simulink model "pendule"  (R2012b)
settings: Solver=ode45  StartTime=0.0  StopTime=10  MaxStep=10  RelTol=1e-3  AbsTol=1e-3
settings Model: ExtModeTrigMode=oneshot  ExtModeArmWhenConnect=off  Creator=ArbenCela  LastModifiedBy=lalinden
settings DataIOCC: LimitDataPoints=off  SignalLoggingSaveFormat=ModelDataLogs  SaveOutput=off  SaveTime=off
settings OptimizationCC: BlockReduction=off  BooleanDataType=off  ExpressionDepthLimit=128  InitFltsAndDblsToZero=on
settings DebuggingCC: SaveWithParameterizedLinksMsg=none  SignalResolutionControl=TryResolveAllWithWarning  SolverPrmCheckMsg=none  MultiTaskDSMMsg=warning  MultiTaskCondExecSysMsg=none  FcnCallInpInsideContextMsg=UseLocalSettings  StateNameClashWarn=none  StrictBusMsg=None
settings HardwareCC: TargetUnknown=on
settings RTWCC: IncludeERTFirstTime=on
settings CodeAppCC: CustomSymbolStrType=$N$R$M_T  InternalIdentifier=Shortened
settings GRTTargetCC: TargetFcnLib=ansi_tfl_tmw.mat  CodeReplacementLibrary=None  CombineOutputUpdateFcns=off  CPPClassGenCompliant=on  GRTInterface=on

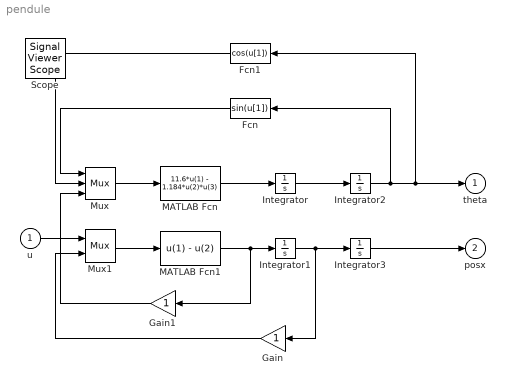
== system pendule ==
  u : Inport
  Fcn : Fcn
  Fcn1 : Fcn  Expr=cos(u[1])
  Gain : Gain  SaturateOnIntegerOverflow=on  OutDataTypeStr=Inherit: Same as input  ParamDataTypeStr=Inherit: Same as input
  Gain1 : Gain  SaturateOnIntegerOverflow=on  OutDataTypeStr=Inherit: Same as input  ParamDataTypeStr=Inherit: Same as input
  Integrator{,1..3} (4 alike) : Integrator
  MATLAB Fcn : MATLABFcn  MATLABFcn=11.6*u(1) - 1.184*u(2)*u(3)  OutputDimensions=1
  MATLAB Fcn1 : MATLABFcn  MATLABFcn=u(1) - u(2)  OutputDimensions=1
  Mux : Mux  Inputs=3
  Mux1 : Mux  Inputs=2
  theta : Outport
  posx : Outport  Port=2
  Scope : SignalViewerScope  IOType=viewer  RefreshTime=0.035000
  wires:
  u/1 -> Mux1/1
  Gain/1 -> Mux1/2
  Gain1/1 -> Mux/3
  MATLAB Fcn1/1 -> Gain1/1, Integrator1/1
  MATLAB Fcn/1 -> Integrator/1
  Mux/1 -> MATLAB Fcn/1
  Mux1/1 -> MATLAB Fcn1/1
  Fcn1/1 -> Mux/2
  Fcn/1 -> Mux/1
  Integrator2/1 -> Fcn1/1, theta/1, Fcn/1
  Integrator1/1 -> Gain/1, Integrator3/1
  Integrator/1 -> Integrator2/1
  Integrator3/1 -> posx/1
